simulink model "obs_reduced"  (R2022a)
settings: Solver=VariableStepAuto  StartTime=0.0  StopTime=3  RelTol=1e-3
values from neighbouring files (symbols this model uses):
  A = [0 0 0 1 0 0 ... (first row only)    [main.m]
  Aroi = inv(Aro)    [main.m]
  B = [0 0 ... (first row only)    [main.m]
  C = [1 0 0 0 0 0 ... (first row only)    [main.m]
  D1 = [-3.6,0,0 ... (first row only)    [main.m]
  Eo = Tr*B    [main.m]
  Go = eye(3)    [main.m]
  klqr2 = real(inv(R)*B'*P2)    [main.m]
  x0 = [0.2 -0.1 0.15 -1 0.8 0]'    [main.m]
settings Model: Creator=wyton  LastModifiedBy=dzsgy
settings SolverCC: AlgebraicLoopSolver=TrustRegion
settings DebuggingCC: UnconnectedInputMsg=warning  UnconnectedOutputMsg=warning  UnconnectedLineMsg=warning  SFMachineParentedDataDiag=warning

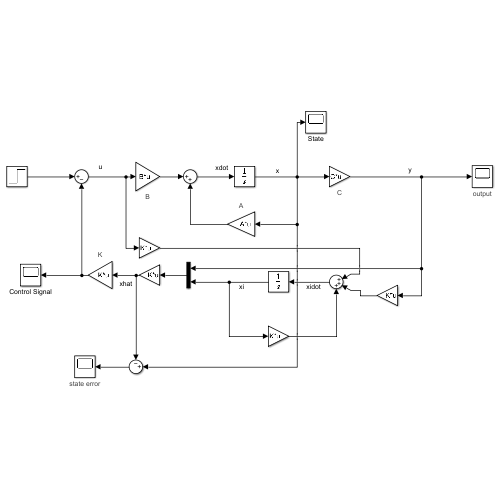
[thumbnail: Simulink's stored preview of the top-level diagram]
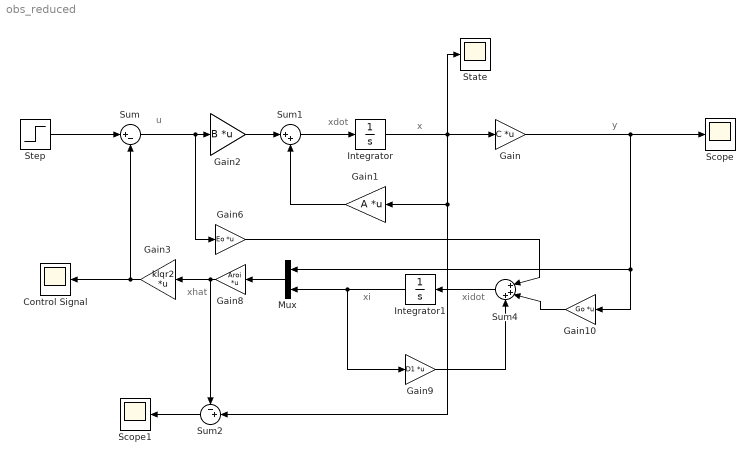
== system obs_reduced ==
  note: xi
  note: xidot
  note: y
  note: xhat
  note: u
  note: xdot
  note: x
  Control Signal : Scope
  Gain : Gain  Gain=C  Multiplication=Matrix(K*u)
      settings: AttributesFormatString=C
  Gain1 : Gain  Gain=A  Multiplication=Matrix(K*u)
      settings: AttributesFormatString=A
  Gain10 : Gain  Gain=Go  Multiplication=Matrix(K*u)
  Gain2 : Gain  Tag=B  Gain=B  Multiplication=Matrix(K*u)
      settings: AttributesFormatString=B
  Gain3 : Gain  Gain=klqr2  Multiplication=Matrix(K*u)
      settings: AttributesFormatString=K
  Gain6 : Gain  Gain=Eo  Multiplication=Matrix(K*u)
  Gain8 : Gain  Gain=Aroi  Multiplication=Matrix(K*u)
  Gain9 : Gain  Gain=D1  Multiplication=Matrix(K*u)
  Integrator : Integrator  InitialCondition=x0
  Integrator1 : Integrator
  Mux : Mux  Inputs=2
  Scope : Scope
      settings: AttributesFormatString=output
  Scope1 : Scope
      settings: AttributesFormatString=state error
  State : Scope
  Step : Step  Time=0  After=0  SampleTime=0
  Sum : Sum  Inputs=|+-
  Sum1 : Sum  Inputs=|++
  Sum2 : Sum  Inputs=-+|
  Sum4 : Sum  Inputs=|+++
  wires:
  Step/1 -> Sum/1
  Sum/1 -> Gain6/1, Gain2/1
  Sum1/1 -> Integrator/1
  Gain2/1 -> Sum1/1
  Integrator/1 -> State/1, Gain1/1, Sum2/2, Gain/1
  Gain1/1 -> Sum1/2
  Gain/1 -> Gain10/1, Mux/1, Scope/1
  Gain3/1 -> Control Signal/1, Sum/2
  Gain8/1 -> Sum2/1, Gain3/1
  Mux/1 -> Gain8/1
  Integrator1/1 -> Gain9/1, Mux/2
  Sum4/1 -> Integrator1/1
  Gain9/1 -> Sum4/3
  Gain10/1 -> Sum4/2
  Gain6/1 -> Sum4/1
  Sum2/1 -> Scope1/1
